simulink library "DKE_Library"  (R2018b)
settings: Solver=VariableStepAuto  StartTime=0.0  StopTime=10.0  RelTol=1e-3
undefined symbols (not defined in the file): dke, ENV, eta_panel, GM, GM_EARTH, Id, N_surf, P0_Sun, q0, r0, req_dke, RW, S_panels, S_surf, SC, v0, vf, w0, ww0, x0
libraries: MATH_library x18, ENV_Library x13, $bdroot x8, simulink x2, sharedtransform x1
(part 2 of 2)

== system DKE_Library/Attitude Dynamics - No Wheels/Derivatives/Quaternion Dynamics/Ω Matrix ==
  ω : Inport
  Add : Sum  Inputs=+++
  Demux : Demux  Outputs=3
  Gain1 : Gain  Gain=[0 0 -1 0; 0 0 0 1; 1 0 0 0; 0 -1 0 0]
  Gain3 : Gain  Gain=[0 1 0 0; -1 0 0 0; 0 0 0 1; 0 0 -1 0]
  Gain4 : Gain  Gain=[0 0 0 1; 0 0 1 0; 0 -1 0 0; -1 0 0 0]
  Ω : Outport  VectorParamsAs1DForOutWhenUnconnected=off
  wires:
  ω/1 -> Demux/1
  Gain1/1 -> Add/2
  Gain3/1 -> Add/3
  Gain4/1 -> Add/1
  Demux/2 -> Gain1/1
  Demux/3 -> Gain3/1
  Add/1 -> Ω/1
  Demux/1 -> Gain4/1
